simulink model "untitled"  (R2023b)
settings: Solver=VariableStepAuto  StartTime=0.0  StopTime=10.0  RelTol=1e-3
settings Model: Creator=CL605_08  LastModifiedBy=CL605_08

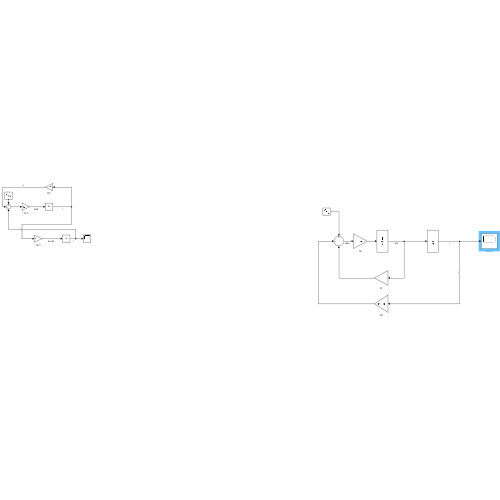
[thumbnail: Simulink's stored preview of the top-level diagram]
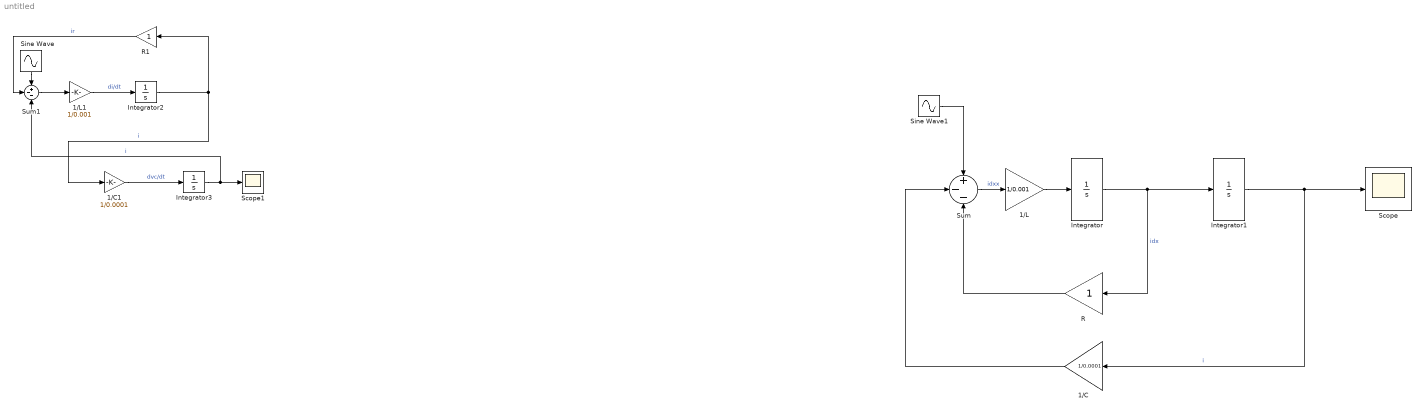
== system untitled ==
  1/C : Gain  Gain=1/0.0001
  1/C1 : Gain  Gain=1/0.0001
  1/L : Gain  Gain=1/0.001
  1/L1 : Gain  Gain=1/0.001
  Integrator{,1..3} (4 alike) : Integrator
  R : Gain
  R1 : Gain
  Scope : Scope
  Scope1 : Scope
  Sine Wave : Sin  Amplitude=2  Frequency=62.5  SampleTime=0
  Sine Wave1 : Sin  Amplitude=2  Frequency=62.5  SampleTime=0
  Sum : Sum  Inputs=+--
  Sum1 : Sum  Inputs=+--
  wires:
  Sum/1 -> 1/L/1  "idxx"
  Integrator/1 -> R/1, Integrator1/1  "idx"
  Integrator1/1 -> 1/C/1, Scope/1  "i"
  R/1 -> Sum/3
  1/C/1 -> Sum/2
  Sine Wave1/1 -> Sum/1
  1/L/1 -> Integrator/1
  1/L1/1 -> Integrator2/1  "di/dt"
  Sum1/1 -> 1/L1/1
  1/C1/1 -> Integrator3/1  "dvc/dt"
  Integrator2/1 -> R1/1, 1/C1/1  "i"
  Integrator3/1 -> Sum1/3, Scope1/1  "i"
  R1/1 -> Sum1/2  "ir"
  Sine Wave/1 -> Sum1/1
